simulink model "Controllo_din_inversa_OPERATIVO"  (R2023b)
settings: Solver=VariableStepAuto  StartTime=0.0  StopTime=10.0  RelTol=1e-3
undefined symbols (not defined in the file): b11, b12, b22, b_1, b_2, d_1, d_2, delta_b11, delta_b12, F1, F2, g1_1, g1_2, g2, gr, h, I_1, I_2, Im_1, Im_2, KD, KP, kr_1, kr_2, kt_1, kt_2, kv_1, kv_2, L_1, L_2, m_1, m_2, mm_2, qc_dd, Ra_1, Ra_2, tc, th1_0, th1d_0, th2_0, th2d_0
settings Model: Creator=Tommaso Savino  LastModifiedBy=Francesco_Savino

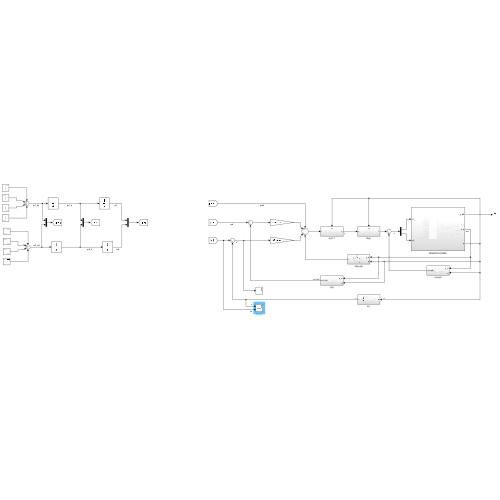
[thumbnail: Simulink's stored preview of the top-level diagram]
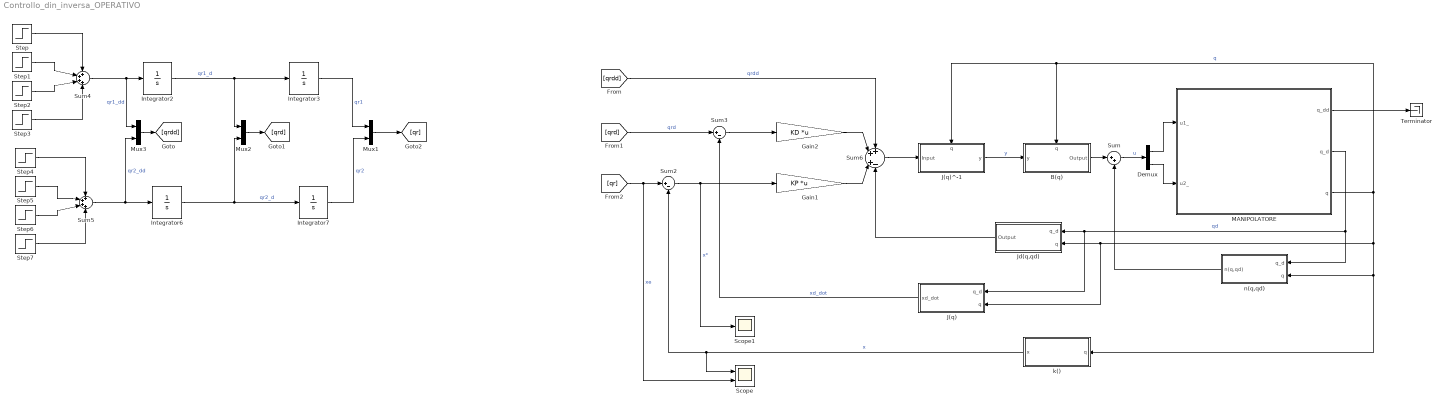
== system Controllo_din_inversa_OPERATIVO ==
  B(q) : Subsystem
      settings: PortSchema="{\"entries\":[{\"content\":{\"sides\":[{\"content\":{\"connectorIds\":[\"In1\"]},\"type\":\"ConnectorPlacement.EquallySpacedRectSide\",\"uuid\":\"bbc9a513-2d37-434b-b23e-4dc451bcd22f\"},{\"content\":{\"connectorIds\":[\"Out1\"],\"side\":\"RIGHT\"},\"type\":\"ConnectorPlacement.EquallySpacedRectSide\",\"uuid\":\"d2460926-2f38-42cc-bb12-745d42388ece\"},{\"content\":{\"connectorIds\":[\"In2\"],\"side\":\"TOP\"},\"type\":\"ConnectorPlacement.EquallySpacedRectSide\",\"uuid\":\"aeb2248f-89a4-438a-8c64-2b1b8cff1973\"}]},\"type\":\"ConnectorPlacement.EquallySpacedConnector\",\"uuid\":\"6c3609d5-174b-43d9-96a5-1a42f99e2581\"}],\"packageUris\":[\"http://schema.mathworks.com/mf0/Connector/R2020b\"],\"version\":\"1.0\"}"
  Demux : Demux  Outputs=2
  Gain1 : Gain  Gain=KP  Multiplication=Matrix(K*u) (u vector)
  Gain2 : Gain  Gain=KD  Multiplication=Matrix(K*u) (u vector)
  Integrator{2..3,6..7} (4 alike) : Integrator
  J(q) : Subsystem
  J(q)^-1 : Subsystem
      settings: PortSchema="{\"entries\":[{\"content\":{\"sides\":[{\"content\":{\"connectorIds\":[\"In1\"]},\"type\":\"ConnectorPlacement.EquallySpacedRectSide\",\"uuid\":\"515bc5bd-4876-4961-a034-aea24abec9fd\"},{\"content\":{\"connectorIds\":[\"Out1\"],\"side\":\"RIGHT\"},\"type\":\"ConnectorPlacement.EquallySpacedRectSide\",\"uuid\":\"1d0a2c9d-18e4-4c5e-8091-1d13b4417a11\"},{\"content\":{\"connectorIds\":[\"In2\"],\"side\":\"TOP\"},\"type\":\"ConnectorPlacement.EquallySpacedRectSide\",\"uuid\":\"0118a193-b043-45d6-8e6e-329b2fdaf764\"}]},\"type\":\"ConnectorPlacement.EquallySpacedConnector\",\"uuid\":\"91b6c9cd-145b-46ff-a2ec-d4d3d0262bff\"}],\"packageUris\":[\"http://schema.mathworks.com/mf0/Connector/R2020b\"],\"version\":\"1.0\"}"
  Jd(q,qd) : Subsystem
  MANIPOLATORE : Subsystem
  Mux1 : Mux  Inputs=2
  Mux2 : Mux  Inputs=2
  Mux3 : Mux  Inputs=2
  Scope : Scope  NumInputPorts=2
  Scope1 : Scope
  Step : Step  Time=0  After=qc_dd  SampleTime=0
  Step1 : Step  Time=tc  After=-qc_dd  SampleTime=0
  Step2 : Step  Time=tf-tc  After=-qc_dd  SampleTime=0
  Step3 : Step  Time=tf  After=qc_dd  SampleTime=0
  Step4 : Step  Time=0  After=qc_dd  SampleTime=0
  Step5 : Step  Time=tc  After=-qc_dd  SampleTime=0
  Step6 : Step  Time=tf-tc  After=-qc_dd  SampleTime=0
  Step7 : Step  Time=tf  After=qc_dd  SampleTime=0
  Sum : Sum  Inputs=|++
  Sum2 : Sum  Inputs=|+-
  Sum3 : Sum  Inputs=|+-
  Sum4 : Sum  Inputs=4
  Sum5 : Sum  Inputs=4
  Sum6 : Sum  Inputs=++|+-
  Terminator : Terminator
  k() : Subsystem
  n(q,qd) : Subsystem
  wires:
  Sum2/1 -> Scope1/1, Gain1/1  "x*"
  n(q,qd)/1(n(q,qd)) -> Sum/2
  Sum/1 -> Demux/1  "u"
  Gain1/1 -> Sum6/3
  MANIPOLATORE/2(q_d) -> n(q,qd)/1(q_d), J(q)/1(q_d), Jd(q,qd)/1(q_d)  "qd"
  Demux/2 -> MANIPOLATORE/2(u2_)
  MANIPOLATORE/1(q_dd) -> Terminator/1
  Demux/1 -> MANIPOLATORE/1(u1_)
  MANIPOLATORE/3(q) -> J(q)^-1/2(q), B(q)/2(q), J(q)/2(q), Jd(q,qd)/2(q), k()/1(q), n(q,qd)/2(q)  "q"
  Gain2/1 -> Sum6/2
  [qrdd] -> Sum6/1  "qrdd"
  Sum3/1 -> Gain2/1
  Step1/1 -> Sum4/2
  Step3/1 -> Sum4/4
  Step/1 -> Sum4/1
  Sum4/1 -> Mux3/1, Integrator2/1  "qr1_dd"
  Integrator2/1 -> Mux2/1, Integrator3/1  "qr1_d"
  Step2/1 -> Sum4/3
  Integrator3/1 -> Mux1/1  "qr1"
  Step7/1 -> Sum5/4
  Step6/1 -> Sum5/3
  Integrator6/1 -> Mux2/2, Integrator7/1  "qr2_d"
  Step5/1 -> Sum5/2
  Step4/1 -> Sum5/1
  Integrator7/1 -> Mux1/2  "qr2"
  Sum5/1 -> Mux3/2, Integrator6/1  "qr2_dd"
  Mux3/1 -> [qrdd]
  Mux2/1 -> [qrd]
  Mux1/1 -> [qr]
  [qrd] -> Sum3/1  "qrd"
  Sum6/1 -> J(q)^-1/1(Input)
  B(q)/1(Output) -> Sum/1
  J(q)/1(xd_dot) -> Sum3/2  "xd_dot"
  J(q)^-1/1(y) -> B(q)/1(y)  "y"
  [qr] -> Scope/2, Sum2/1  "xe"
  k()/1(x) -> Scope/1, Sum2/2  "x"
  Jd(q,qd)/1(Output) -> Sum6/4

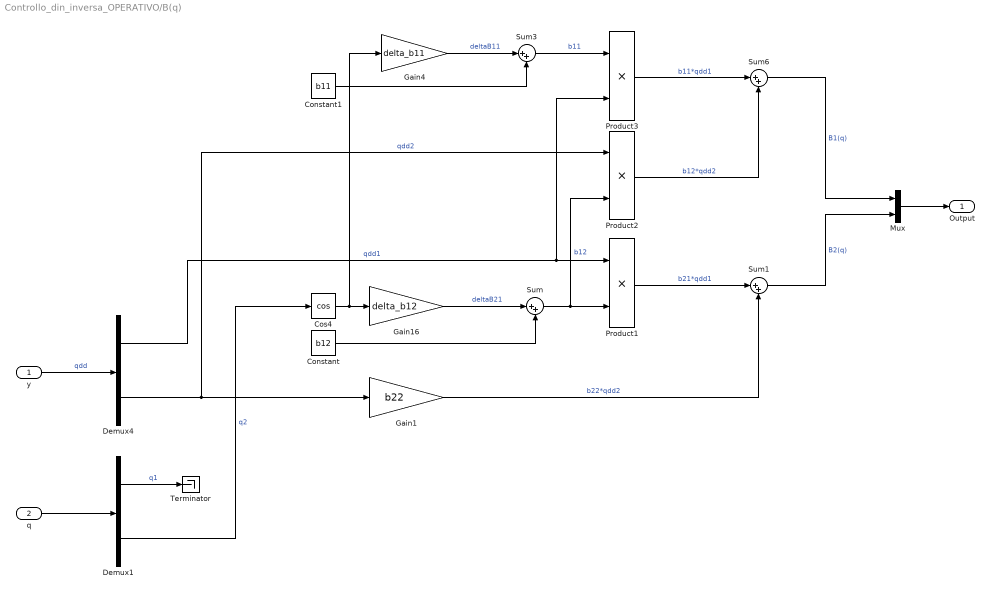
== system Controllo_din_inversa_OPERATIVO/B(q) ==
  y : Inport
  q : Inport  Port=2
  Constant : Constant  Value=b12
  Constant1 : Constant  Value=b11
  Cos4 : Trigonometry  Operator=cos
  Demux1 : Demux  Outputs=2
  Demux4 : Demux  Outputs=2
  Gain1 : Gain  Gain=b22
  Gain16 : Gain  Gain=delta_b12
  Gain4 : Gain  Gain=delta_b11
  Mux : Mux  Inputs=2
  Product1 : Product
  Product2 : Product
  Product3 : Product
  Sum{,1,3,6} (4 alike) : Sum  Inputs=|++
  Terminator : Terminator
  Output : Outport
  wires:
  Sum6/1 -> Mux/1  "B1(q)"
  Sum3/1 -> Product3/1  "b11"
  Constant1/1 -> Sum3/2
  Sum1/1 -> Mux/2  "B2(q)"
  Gain1/1 -> Sum1/2  "b22*qdd2"
  Product1/1 -> Sum1/1  "b21*qdd1"
  Sum/1 -> Product2/2, Product1/2  "b12"
  Constant/1 -> Sum/2
  Demux1/2 -> Cos4/1  "q2"
  Demux1/1 -> Terminator/1  "q1"
  Demux4/2 -> Product2/1, Gain1/1  "qdd2"
  Gain4/1 -> Sum3/1  "deltaB11"
  Demux4/1 -> Product1/1, Product3/2  "qdd1"
  Product3/1 -> Sum6/1  "b11*qdd1"
  Product2/1 -> Sum6/2  "b12*qdd2"
  Cos4/1 -> Gain4/1, Gain16/1
  Gain16/1 -> Sum/1  "deltaB21"
  y/1 -> Demux4/1  "qdd"
  q/1 -> Demux1/1
  Mux/1 -> Output/1

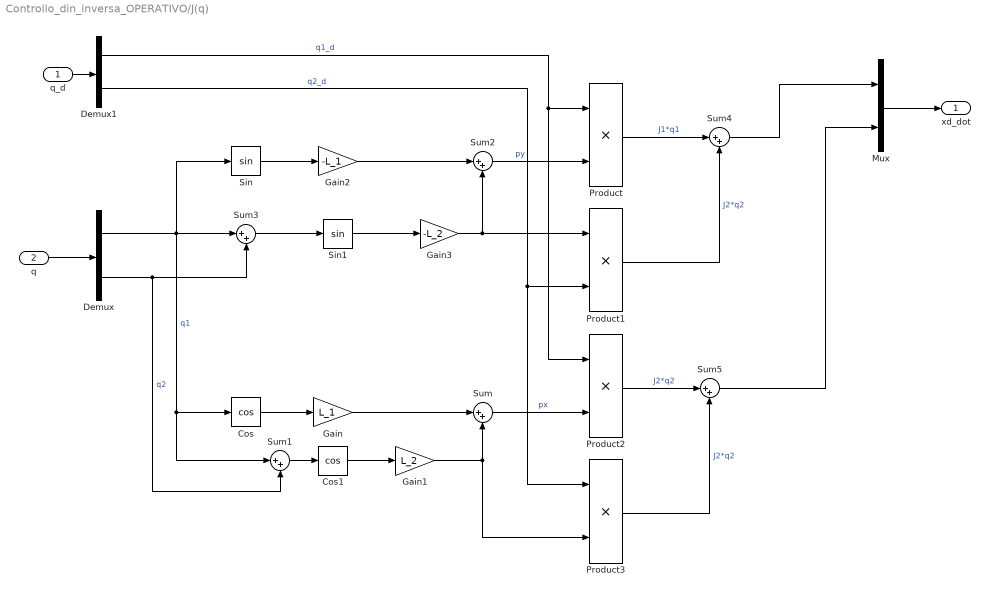
== system Controllo_din_inversa_OPERATIVO/J(q) ==
  q_d : Inport
  q : Inport  Port=2
  Cos : Trigonometry  Operator=cos
  Cos1 : Trigonometry  Operator=cos
  Demux : Demux  Outputs=2
  Demux1 : Demux  Outputs=2
  Gain : Gain  Gain=L_1
  Gain1 : Gain  Gain=L_2
  Gain2 : Gain  Gain=-L_1
  Gain3 : Gain  Gain=-L_2
  Mux : Mux  Inputs=2
  Product{,1..3} (4 alike) : Product
  Sin : Trigonometry
  Sin1 : Trigonometry
  Sum{,1..5} (6 alike) : Sum  Inputs=|++
  xd_dot : Outport
  wires:
  Sum3/1 -> Sin1/1
  Sin1/1 -> Gain3/1
  Sin/1 -> Gain2/1
  Sum2/1 -> Product/2  "py"
  Gain2/1 -> Sum2/1
  Gain3/1 -> Product1/1, Sum2/2
  q/1 -> Demux/1
  q_d/1 -> Demux1/1
  Demux1/1 -> Product2/1, Product/1  "q1_d"
  Product/1 -> Sum4/1  "J1*q1"
  Sum4/1 -> Mux/1
  Mux/1 -> xd_dot/1
  Demux1/2 -> Product3/1, Product1/2  "q2_d"
  Product1/1 -> Sum4/2  "J2*q2"
  Gain/1 -> Sum/1
  Cos1/1 -> Gain1/1
  Demux/1 -> Sum3/1, Cos/1, Sum1/1, Sin/1  "q1"
  Demux/2 -> Sum1/2, Sum3/2  "q2"
  Gain1/1 -> Product3/2, Sum/2
  Cos/1 -> Gain/1
  Sum1/1 -> Cos1/1
  Sum/1 -> Product2/2  "px"
  Product2/1 -> Sum5/1  "J2*q2"
  Product3/1 -> Sum5/2  "J2*q2"
  Sum5/1 -> Mux/2

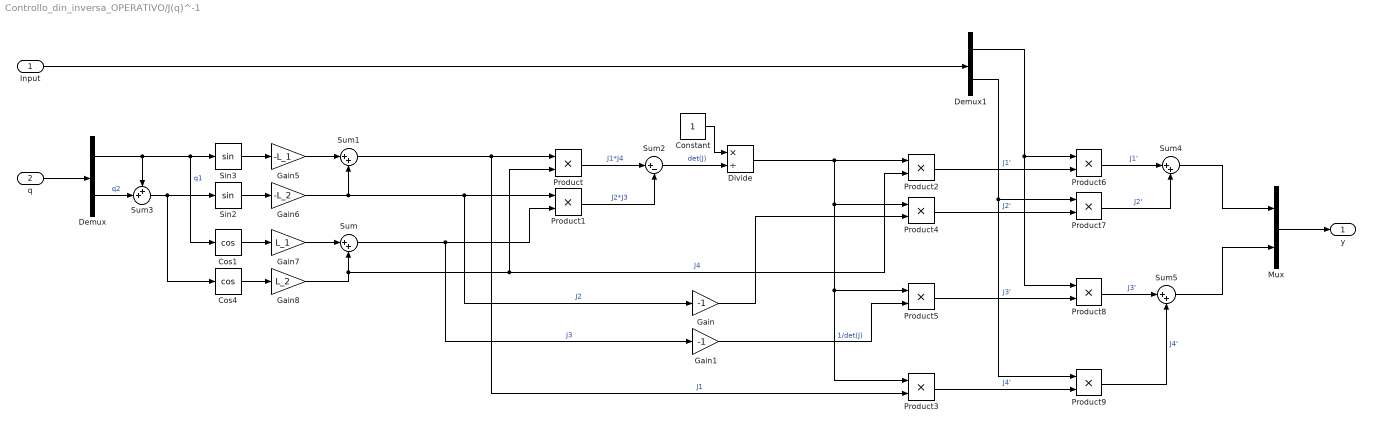
== system Controllo_din_inversa_OPERATIVO/J(q)^-1 ==
  Input : Inport
  q : Inport  Port=2
  Constant : Constant
  Cos1 : Trigonometry  Operator=cos
  Cos4 : Trigonometry  Operator=cos
  Demux : Demux  Outputs=2
  Demux1 : Demux  Outputs=2
  Divide : Product  Inputs=*/
  Gain : Gain  Gain=-1
  Gain1 : Gain  Gain=-1
  Gain5 : Gain  Gain=-L_1
  Gain6 : Gain  Gain=-L_2
  Gain7 : Gain  Gain=L_1
  Gain8 : Gain  Gain=L_2
  Mux : Mux  Inputs=2
  Product{,1..9} (10 alike) : Product
  Sin2 : Trigonometry
  Sin3 : Trigonometry
  Sum{,1,4..5} (4 alike) : Sum  Inputs=|++
  Sum2 : Sum  Inputs=|+-
  Sum3 : Sum  Inputs=++|
  y : Outport
  wires:
  Mux/1 -> y/1
  Input/1 -> Demux1/1
  Sin3/1 -> Gain5/1
  Demux/2 -> Sum3/2  "q2"
  Sum3/1 -> Sin2/1, Cos4/1
  Sin2/1 -> Gain6/1
  Gain7/1 -> Sum/1
  Gain5/1 -> Sum1/1
  Demux/1 -> Sin3/1, Cos1/1, Sum3/1  "q1"
  q/1 -> Demux/1
  Gain8/1 -> Product2/2, Product/2, Sum/2  "J4"
  Gain6/1 -> Gain/1, Product1/1, Sum1/2  "J2"
  Sum/1 -> Product1/2, Gain1/1  "J3"
  Sum1/1 -> Product3/2, Product/1  "J1"
  Cos1/1 -> Gain7/1
  Cos4/1 -> Gain8/1
  Product/1 -> Sum2/1  "J1*J4"
  Product1/1 -> Sum2/2  "J2*J3"
  Sum2/1 -> Divide/2  "det(J)"
  Constant/1 -> Divide/1
  Divide/1 -> Product5/1, Product3/1, Product4/1, Product2/1  "1/det(J)"
  Product2/1 -> Product6/2  "J1'"
  Product3/1 -> Product9/2  "J4'"
  Gain/1 -> Product4/2
  Product4/1 -> Product7/2  "J2'"
  Gain1/1 -> Product5/2
  Product5/1 -> Product8/2  "J3'"
  Product8/1 -> Sum5/1  "J3'"
  Product9/1 -> Sum5/2  "J4'"
  Product6/1 -> Sum4/1  "J1'"
  Product7/1 -> Sum4/2  "J2'"
  Sum4/1 -> Mux/1
  Sum5/1 -> Mux/2
  Demux1/1 -> Product8/1, Product6/1
  Demux1/2 -> Product9/1, Product7/1

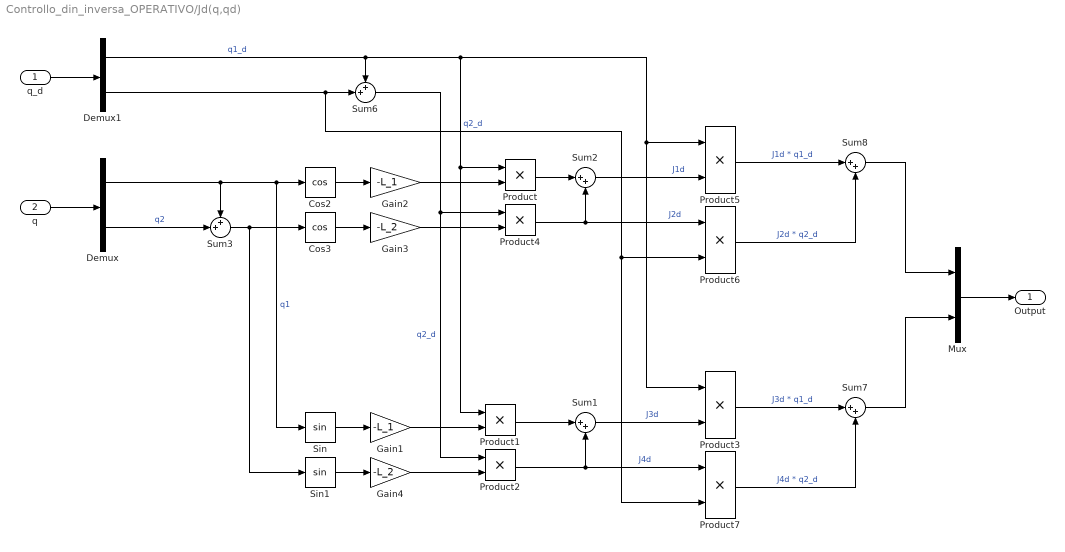
== system Controllo_din_inversa_OPERATIVO/Jd(q,qd) ==
  q_d : Inport
  q : Inport  Port=2
  Cos2 : Trigonometry  Operator=cos
  Cos3 : Trigonometry  Operator=cos
  Demux : Demux  Outputs=2
  Demux1 : Demux  Outputs=2
  Gain1 : Gain  Gain=-L_1
  Gain2 : Gain  Gain=-L_1
  Gain3 : Gain  Gain=-L_2
  Gain4 : Gain  Gain=-L_2
  Mux : Mux  Inputs=2
  Product{,1..7} (8 alike) : Product
  Sin : Trigonometry
  Sin1 : Trigonometry
  Sum{1..2,7..8} (4 alike) : Sum  Inputs=|++
  Sum3 : Sum  Inputs=++|
  Sum6 : Sum  Inputs=++|
  Output : Outport
  wires:
  Mux/1 -> Output/1
  q_d/1 -> Demux1/1
  q/1 -> Demux/1
  Gain3/1 -> Product4/2
  Gain2/1 -> Product/2
  Cos2/1 -> Gain2/1
  Cos3/1 -> Gain3/1
  Product/1 -> Sum2/1
  Sum3/1 -> Sin1/1, Cos3/1
  Product4/1 -> Product6/1, Sum2/2  "J2d"
  Sum6/1 -> Product2/1, Product4/1  "q2_d"
  Sum2/1 -> Product5/2  "J1d"
  Product5/1 -> Sum8/1  "J1d * q1_d"
  Product1/1 -> Sum1/1
  Demux1/2 -> Product7/2, Product6/2, Sum6/2  "q2_d"
  Sin/1 -> Gain1/1
  Demux/2 -> Sum3/2  "q2"
  Demux/1 -> Sin/1, Cos2/1, Sum3/1  "q1"
  Demux1/1 -> Product3/1, Product5/1, Product1/1, Product/1, Sum6/1  "q1_d"
  Sum1/1 -> Product3/2  "J3d"
  Gain4/1 -> Product2/2
  Product3/1 -> Sum7/1  "J3d * q1_d"
  Sin1/1 -> Gain4/1
  Gain1/1 -> Product1/2
  Product2/1 -> Product7/1, Sum1/2  "J4d"
  Product6/1 -> Sum8/2  "J2d * q2_d"
  Sum8/1 -> Mux/1
  Product7/1 -> Sum7/2  "J4d * q2_d"
  Sum7/1 -> Mux/2

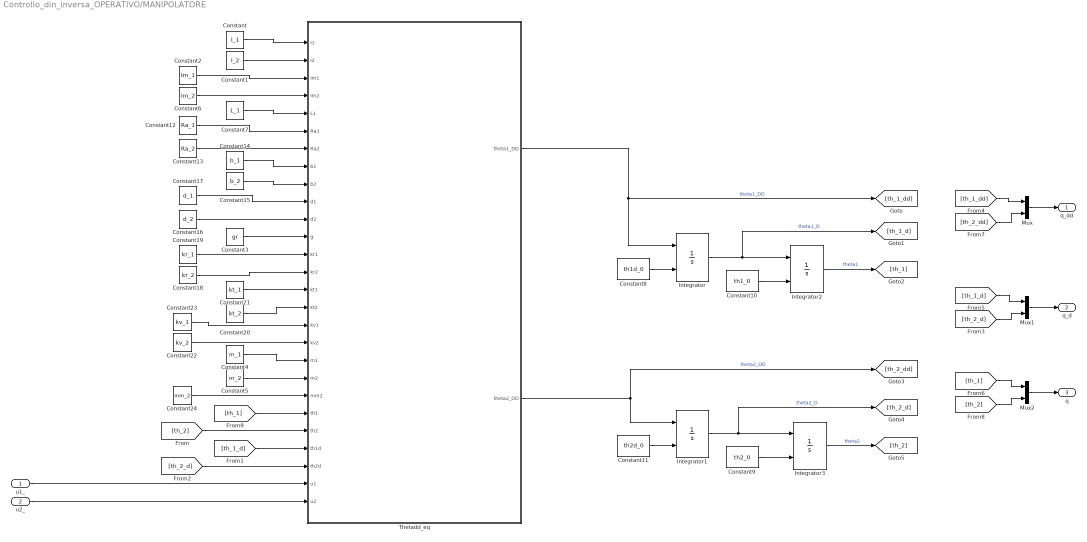
== system Controllo_din_inversa_OPERATIVO/MANIPOLATORE ==
  u1_ : Inport
  u2_ : Inport  Port=2
  Constant : Constant  Value=I_1
  Constant1 : Constant  Value=I_2
  Constant10 : Constant  Value=th1_0
  Constant11 : Constant  Value=th2d_0
  Constant12 : Constant  Value=Ra_1
  Constant13 : Constant  Value=Ra_2
  Constant14 : Constant  Value=b_1
  Constant15 : Constant  Value=b_2
  Constant16 : Constant  Value=d_2
  Constant17 : Constant  Value=d_1
  Constant18 : Constant  Value=kr_2
  Constant19 : Constant  Value=kr_1
  Constant2 : Constant  Value=Im_1
  Constant20 : Constant  Value=kt_2
  Constant21 : Constant  Value=kt_1
  Constant22 : Constant  Value=kv_2
  Constant23 : Constant  Value=kv_1
  Constant24 : Constant  Value=mm_2
  Constant3 : Constant  Value=gr
  Constant4 : Constant  Value=m_1
  Constant5 : Constant  Value=m_2
  Constant6 : Constant  Value=Im_2
  Constant7 : Constant  Value=L_1
  Constant8 : Constant  Value=th1d_0
  Constant9 : Constant  Value=th2_0
  Integrator{,1..3} (4 alike) : Integrator  InitialConditionSource=external
  Mux : Mux  Inputs=2
  Mux1 : Mux  Inputs=2
  Mux2 : Mux  Inputs=2
  Thetadd_eq : MATLAB Function  TreatAsAtomicUnit=on
  q_dd : Outport
  q_d : Outport  Port=2
  q : Outport  Port=3
  wires:
  Constant9/1 -> Integrator3/2
  Constant1/1 -> Thetadd_eq/2(I2)
  [th_2] -> Thetadd_eq/23(th2)
  Thetadd_eq/2(theta2_DD) -> Integrator1/1, [th_2_dd]  "theta2_DD"
  Constant5/1 -> Thetadd_eq/20(m2)
  Constant7/1 -> Thetadd_eq/5(L1)
  Constant3/1 -> Thetadd_eq/12(g)
  Thetadd_eq/1(theta1_DD) -> Integrator/1, [th_1_dd]  "theta1_DD"
  [th_1_d] -> Thetadd_eq/24(th1d)
  Integrator3/1 -> [th_2]  "theta2"
  Constant/1 -> Thetadd_eq/1(I1)
  Integrator2/1 -> [th_1]  "theta1"
  Constant2/1 -> Thetadd_eq/3(Im1)
  Integrator/1 -> [th_1_d], Integrator2/1  "theta1_D"
  Constant10/1 -> Integrator2/2
  Constant11/1 -> Integrator1/2
  Integrator1/1 -> [th_2_d], Integrator3/1  "theta2_D"
  Constant4/1 -> Thetadd_eq/19(m1)
  Constant8/1 -> Integrator/2
  [th_2_d] -> Thetadd_eq/25(th2d)
  Constant6/1 -> Thetadd_eq/4(Im2)
  u1_/1 -> Thetadd_eq/26(u1)
  u2_/1 -> Thetadd_eq/27(u2)
  [th_1_dd] -> Mux/1
  [th_2_dd] -> Mux/2
  Mux/1 -> q_dd/1
  [th_1_d] -> Mux1/1
  [th_2_d] -> Mux1/2
  Mux1/1 -> q_d/1
  [th_1] -> Mux2/1
  [th_2] -> Mux2/2
  Mux2/1 -> q/1
  Constant12/1 -> Thetadd_eq/6(Ra1)
  Constant13/1 -> Thetadd_eq/7(Ra2)
  Constant14/1 -> Thetadd_eq/8(b1)
  Constant15/1 -> Thetadd_eq/9(b2)
  Constant16/1 -> Thetadd_eq/11(d2)
  Constant17/1 -> Thetadd_eq/10(d1)
  Constant19/1 -> Thetadd_eq/13(kr1)
  Constant18/1 -> Thetadd_eq/14(kr2)
  Constant21/1 -> Thetadd_eq/15(kt1)
  Constant20/1 -> Thetadd_eq/16(kt2)
  Constant23/1 -> Thetadd_eq/17(kv1)
  Constant22/1 -> Thetadd_eq/18(kv2)
  Constant24/1 -> Thetadd_eq/21(mm2)
  [th_1] -> Thetadd_eq/22(th1)

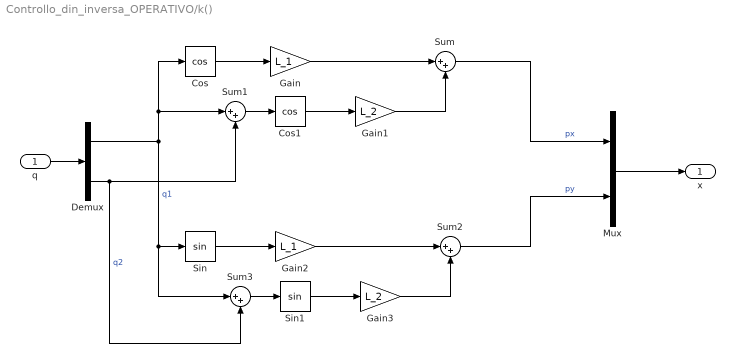
== system Controllo_din_inversa_OPERATIVO/k() ==
  q : Inport
  Cos : Trigonometry  Operator=cos
  Cos1 : Trigonometry  Operator=cos
  Demux : Demux  Outputs=2
  Gain : Gain  Gain=L_1
  Gain1 : Gain  Gain=L_2
  Gain2 : Gain  Gain=L_1
  Gain3 : Gain  Gain=L_2
  Mux : Mux  Inputs=2
  Sin : Trigonometry
  Sin1 : Trigonometry
  Sum{,1..3} (4 alike) : Sum  Inputs=|++
  x : Outport
  wires:
  q/1 -> Demux/1
  Demux/1 -> Sum3/1, Sin/1, Sum1/1, Cos/1  "q1"
  Demux/2 -> Sum1/2, Sum3/2  "q2"
  Cos/1 -> Gain/1
  Gain/1 -> Sum/1
  Sum1/1 -> Cos1/1
  Cos1/1 -> Gain1/1
  Gain1/1 -> Sum/2
  Sum3/1 -> Sin1/1
  Gain3/1 -> Sum2/2
  Sin/1 -> Gain2/1
  Sin1/1 -> Gain3/1
  Gain2/1 -> Sum2/1
  Sum2/1 -> Mux/2  "py"
  Sum/1 -> Mux/1  "px"
  Mux/1 -> x/1

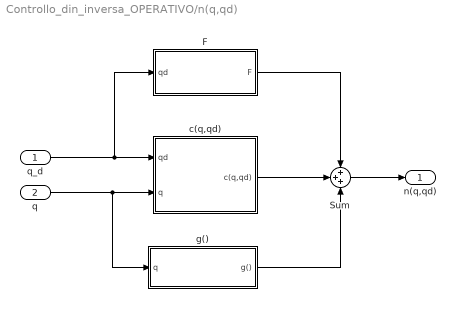
== system Controllo_din_inversa_OPERATIVO/n(q,qd) ==
  q_d : Inport
  q : Inport  Port=2
  F : Subsystem
  Sum : Sum  Inputs=+++
  c(q,qd) : Subsystem
  g() : Subsystem
  n(q,qd) : Outport
  wires:
  F/1(F) -> Sum/1
  q_d/1 -> c(q,qd)/1(qd), F/1(qd)
  Sum/1 -> n(q,qd)/1
  g()/1(g()) -> Sum/3
  c(q,qd)/1(c(q,qd)) -> Sum/2
  q/1 -> c(q,qd)/2(q), g()/1(q)

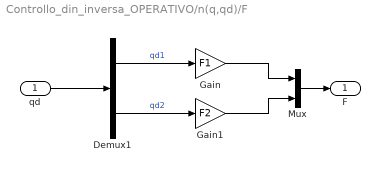
== system Controllo_din_inversa_OPERATIVO/n(q,qd)/F ==
  qd : Inport
  Demux1 : Demux  Outputs=2
  Gain : Gain  Gain=F1
  Gain1 : Gain  Gain=F2
  Mux : Mux  Inputs=2
  F : Outport
  wires:
  Demux1/2 -> Gain1/1  "qd2"
  Gain/1 -> Mux/1
  Mux/1 -> F/1
  Gain1/1 -> Mux/2
  qd/1 -> Demux1/1
  Demux1/1 -> Gain/1  "qd1"

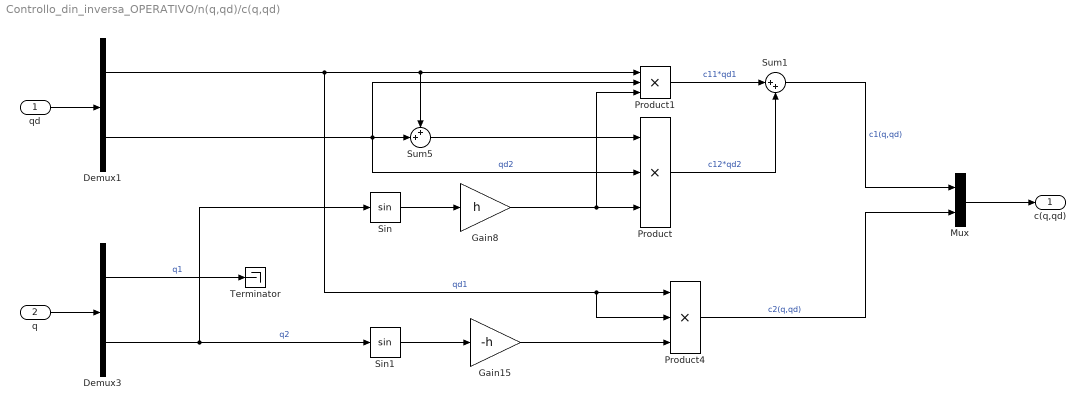
== system Controllo_din_inversa_OPERATIVO/n(q,qd)/c(q,qd) ==
  qd : Inport
  q : Inport  Port=2
  Demux1 : Demux  Outputs=2
  Demux3 : Demux  Outputs=2
  Gain15 : Gain  Gain=-h
  Gain8 : Gain  Gain=h
  Mux : Mux  Inputs=2
  Product : Product  Inputs=3
  Product1 : Product  Inputs=3
  Product4 : Product  Inputs=3
  Sin : Trigonometry
  Sin1 : Trigonometry
  Sum1 : Sum  Inputs=|++
  Sum5 : Sum  Inputs=++|
  Terminator : Terminator
  c(q,qd) : Outport
  wires:
  qd/1 -> Demux1/1
  q/1 -> Demux3/1
  Sin1/1 -> Gain15/1
  Gain15/1 -> Product4/3
  Sum1/1 -> Mux/1  "c1(q,qd)"
  Demux3/2 -> Sin/1, Sin1/1  "q2"
  Sum5/1 -> Product/1
  Product/1 -> Sum1/2  "c12*qd2"
  Demux1/2 -> Sum5/2, Product/2, Product1/2  "qd2"
  Sin/1 -> Gain8/1
  Demux1/1 -> Product4/1, Product4/2, Sum5/1, Product1/1  "qd1"
  Product1/1 -> Sum1/1  "c11*qd1"
  Product4/1 -> Mux/2  "c2(q,qd)"
  Demux3/1 -> Terminator/1  "q1"
  Gain8/1 -> Product/3, Product1/3
  Mux/1 -> c(q,qd)/1

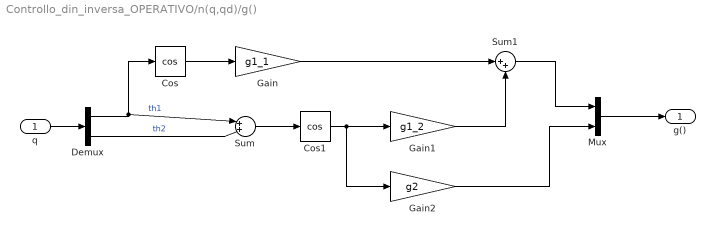
== system Controllo_din_inversa_OPERATIVO/n(q,qd)/g() ==
  q : Inport
  Cos : Trigonometry  Operator=cos
  Cos1 : Trigonometry  Operator=cos
  Demux : Demux  Outputs=2
  Gain : Gain  Gain=g1_1
  Gain1 : Gain  Gain=g1_2
  Gain2 : Gain  Gain=g2
  Mux : Mux  Inputs=2
  Sum : Sum  Inputs=|++|
  Sum1 : Sum  Inputs=|++
  g() : Outport
  wires:
  Gain2/1 -> Mux/2
  Mux/1 -> g()/1
  Sum1/1 -> Mux/1
  Gain1/1 -> Sum1/2
  Gain/1 -> Sum1/1
  Cos1/1 -> Gain1/1, Gain2/1
  Sum/1 -> Cos1/1
  Cos/1 -> Gain/1
  Demux/2 -> Sum/2  "th2"
  Demux/1 -> Sum/1, Cos/1  "th1"
  q/1 -> Demux/1

== matlab function Controllo_din_inversa_OPERATIVO/MANIPOLATORE/Thetadd_eq ==
  data: I1 input; theta1_DD output; I2 input; Im1 input; Im2 input; L1 input; Ra1 input; Ra2 input; b1 input; b2 input; d1 input; d2 input; g input; kr1 input; kr2 input; kt1 input; kt2 input; kv1 input; kv2 input; m1 input; m2 input; mm2 input; th1 input; th2 input; th1d input; th2d input; u1 input; u2 input; theta2_DD output
function [theta1_DD,theta2_DD] = Thetadd_eq(I1,I2,Im1,Im2,L1,Ra1,Ra2,b1,b2,d1,d2,g,kr1,kr2,kt1,kt2,kv1,kv2,m1,m2,mm2,th1,th2,th1d,th2d,u1,u2)
%#codegen

%    This function was generated by the Symbolic Math Toolbox version 23.2.
%    04-Mar-2024 11:53:02

% I1 = complex(I1);  % if required to enforce complex operations
% I2 = complex(I2);  % if required to enforce complex operations
% Im1 = complex(Im1);  % if required to enforce complex operations
% Im2 = complex(Im2);  % if required to enforce complex operations
% L1 = complex(L1);  % if required to enforce complex operations
% Ra1 = complex(Ra1);  % if required to enforce complex operations
% Ra2 = complex(Ra2);  % if required to enforce complex operations
% b1 = complex(b1);  % if required to enforce complex operations
% b2 = complex(b2);  % if required to enforce complex operations
% d1 = complex(d1);  % if required to enforce complex operations
% d2 = complex(d2);  % if required to enforce complex operations
% g = complex(g);  % if required to enforce complex operations
% kr1 = complex(kr1);  % if required to enforce complex operations
% kr2 = complex(kr2);  % if required to enforce complex operations
% kt1 = complex(kt1);  % if required to enforce complex operations
% kt2 = complex(kt2);  % if required to enforce complex operations
% kv1 = complex(kv1);  % if required to enforce complex operations
% kv2 = complex(kv2);  % if required to enforce complex operations
% m1 = complex(m1);  % if required to enforce complex operations
% m2 = complex(m2);  % if required to enforce complex operations
% mm2 = complex(mm2);  % if required to enforce complex operations
% th1 = complex(th1);  % if required to enforce complex operations
% th2 = complex(th2);  % if required to enforce complex operations
% th1d = complex(th1d);  % if required to enforce complex operations
% th2d = complex(th2d);  % if required to enforce complex operations
% u1 = complex(u1);  % if required to enforce complex operations
% u2 = complex(u2);  % if required to enforce complex operations
et1 = I2.*Ra1.*Ra2.*u1-I2.*Ra1.*Ra2.*u2-I2.*Ra1.*Ra2.*b1.*th1d+I2.*Ra1.*Ra2.*b2.*th2d-Im2.*Ra1.*Ra2.*kr2.*u2+Im2.*Ra1.*Ra2.*kr2.^2.*u1+Ra1.*Ra2.*d2.^2.*m2.*u1-Ra1.*Ra2.*d2.^2.*m2.*u2-Ra1.*Ra2.*b1.*d2.^2.*m2.*th1d+Ra1.*Ra2.*b2.*d2.^2.*m2.*th2d-I2.*Ra2.*kr1.^2.*kt1.*kv1.*th1d+I2.*Ra1.*kr2.^2.*kt2.*kv2.*th2d+Im2.*Ra1.*kr2.^3.*kt2.*kv2.*th2d+Im2.*Ra1.*Ra2.*b2.*kr2.*th2d-Im2.*Ra1.*Ra2.*b1.*kr2.^2.*th1d-L1.*Ra1.*Ra2.*d2.^2.*g.*m2.^2.*cos(th1)-I2.*L1.*Ra1.*Ra2.*g.*m2.*cos(th1)-I2.*L1.*Ra1.*Ra2.*g.*mm2.*cos(th1)-I2.*Ra1.*Ra2.*d1.*g.*m1.*cos(th1)-L1.*Ra1.*Ra2.*d2.*m2.*u2.*cos(th2);
et2 = L1.*Ra1.*Ra2.*d2.^3.*m2.^2.*th1d.^2.*sin(th2)+L1.*Ra1.*Ra2.*d2.^3.*m2.^2.*th2d.^2.*sin(th2)-Im2.*Ra2.*kr1.^2.*kr2.^2.*kt1.*kv1.*th1d-Ra2.*d2.^2.*kr1.^2.*kt1.*kv1.*m2.*th1d+Ra1.*d2.^2.*kr2.^2.*kt2.*kv2.*m2.*th2d-Im2.*L1.*Ra1.*Ra2.*g.*kr2.^2.*m2.*cos(th1)-Im2.*L1.*Ra1.*Ra2.*g.*kr2.^2.*mm2.*cos(th1)+I2.*L1.*Ra1.*Ra2.*d2.*m2.*th1d.^2.*sin(th2)+I2.*L1.*Ra1.*Ra2.*d2.*m2.*th2d.^2.*sin(th2)-Im2.*Ra1.*Ra2.*d1.*g.*kr2.^2.*m1.*cos(th1)-L1.*Ra1.*Ra2.*d2.^2.*g.*m2.*mm2.*cos(th1)-Ra1.*Ra2.*d1.*d2.^2.*g.*m1.*m2.*cos(th1)+Im2.*Ra1.*Ra2.*d2.*g.*kr2.*m2.*cos(th1+th2)+L1.*Ra1.*Ra2.*d2.^3.*m2.^2.*th1d.*th2d.*sin(th2).*2.0;
et3 = L1.*Ra1.*Ra2.*d2.^2.*g.*m2.^2.*cos(th1+th2).*cos(th2)+L1.*Ra1.*Ra2.*b2.*d2.*m2.*th2d.*cos(th2)+L1.^2.*Ra1.*Ra2.*d2.^2.*m2.^2.*th1d.^2.*cos(th2).*sin(th2)-Im2.*Ra1.*Ra2.*d2.*g.*kr2.^2.*m2.*cos(th1+th2)+I2.*L1.*Ra1.*Ra2.*d2.*m2.*th1d.*th2d.*sin(th2).*2.0+Im2.*L1.*Ra1.*Ra2.*d2.*kr2.*m2.*th1d.^2.*sin(th2)+L1.*Ra1.*d2.*kr2.^2.*kt2.*kv2.*m2.*th2d.*cos(th2)+Im2.*L1.*Ra1.*Ra2.*d2.*kr2.^2.*m2.*th2d.^2.*sin(th2)+Im2.*L1.*Ra1.*Ra2.*d2.*kr2.^2.*m2.*th1d.*th2d.*sin(th2).*2.0;
et4 = 1.0./(Ra1.*Ra2.*(I1.*I2+I2.*Im2-I2.*Im2.*kr2.*2.0+L1.^2.*d2.^2.*m2.^2+I2.*Im1.*kr1.^2+I1.*Im2.*kr2.^2+I2.*Im2.*kr2.^2+I2.*L1.^2.*m2+I2.*L1.^2.*mm2+I2.*d1.^2.*m1+I1.*d2.^2.*m2+Im2.*d2.^2.*m2-Im2.*d2.^2.*kr2.*m2.*2.0+Im1.*Im2.*kr1.^2.*kr2.^2+Im2.*L1.^2.*kr2.^2.*m2+Im2.*L1.^2.*kr2.^2.*mm2+Im1.*d2.^2.*kr1.^2.*m2+Im2.*d1.^2.*kr2.^2.*m1+Im2.*d2.^2.*kr2.^2.*m2+L1.^2.*d2.^2.*m2.*mm2+d1.^2.*d2.^2.*m1.*m2-L1.^2.*d2.^2.*m2.^2.*cos(th2).^2-Im2.*L1.*d2.*kr2.*m2.*cos(th2).*2.0+Im2.*L1.*d2.*kr2.^2.*m2.*cos(th2).*2.0));
et5 = et1+et2+et3;
theta1_DD = et4.*et5;
if nargout > 1
    et6 = -I1.*Ra1.*Ra2.*u2+I2.*Ra1.*Ra2.*u1-I2.*Ra1.*Ra2.*u2-Im2.*Ra1.*Ra2.*u2-I2.*Ra1.*Ra2.*b1.*th1d+I1.*Ra1.*Ra2.*b2.*th2d+I2.*Ra1.*Ra2.*b2.*th2d+Im2.*Ra1.*Ra2.*b2.*th2d+Im2.*Ra1.*Ra2.*kr2.*u1-Im1.*Ra1.*Ra2.*kr1.^2.*u2-L1.^2.*Ra1.*Ra2.*m2.*u2-L1.^2.*Ra1.*Ra2.*mm2.*u2-Ra1.*Ra2.*d1.^2.*m1.*u2+Ra1.*Ra2.*d2.^2.*m2.*u1-Ra1.*Ra2.*d2.^2.*m2.*u2-Ra1.*Ra2.*b1.*d2.^2.*m2.*th1d+Ra1.*Ra2.*b2.*d1.^2.*m1.*th2d+Ra1.*Ra2.*b2.*d2.^2.*m2.*th2d-I2.*Ra2.*kr1.^2.*kt1.*kv1.*th1d+I1.*Ra1.*kr2.^2.*kt2.*kv2.*th2d+I2.*Ra1.*kr2.^2.*kt2.*kv2.*th2d+Im2.*Ra1.*kr2.^2.*kt2.*kv2.*th2d-Im2.*Ra1.*Ra2.*b1.*kr2.*th1d;
    et7 = Im1.*Ra1.*Ra2.*b2.*kr1.^2.*th2d+L1.^2.*Ra1.*Ra2.*b2.*m2.*th2d+L1.^2.*Ra1.*Ra2.*b2.*mm2.*th2d-L1.*Ra1.*Ra2.*d2.^2.*g.*m2.^2.*cos(th1)+I1.*Ra1.*Ra2.*d2.*g.*m2.*cos(th1+th2)+Im2.*Ra1.*Ra2.*d2.*g.*m2.*cos(th1+th2)-I2.*L1.*Ra1.*Ra2.*g.*m2.*cos(th1)-I2.*L1.*Ra1.*Ra2.*g.*mm2.*cos(th1)-I2.*Ra1.*Ra2.*d1.*g.*m1.*cos(th1)+L1.*Ra1.*Ra2.*d2.*m2.*u1.*cos(th2)-L1.*Ra1.*Ra2.*d2.*m2.*u2.*cos(th2).*2.0-Im2.*Ra2.*kr1.^2.*kr2.*kt1.*kv1.*th1d+L1.*Ra1.*Ra2.*d2.^3.*m2.^2.*th1d.^2.*sin(th2)+L1.^3.*Ra1.*Ra2.*d2.*m2.^2.*th1d.^2.*sin(th2)+L1.*Ra1.*Ra2.*d2.^3.*m2.^2.*th2d.^2.*sin(th2)+Im1.*Ra1.*kr1.^2.*kr2.^2.*kt2.*kv2.*th2d+L1.^2.*Ra1.*kr2.^2.*kt2.*kv2.*m2.*th2d;
    et8 = L1.^2.*Ra1.*kr2.^2.*kt2.*kv2.*mm2.*th2d+L1.^2.*Ra1.*Ra2.*d2.*g.*m2.^2.*cos(th1+th2)-Ra2.*d2.^2.*kr1.^2.*kt1.*kv1.*m2.*th1d+Ra1.*d1.^2.*kr2.^2.*kt2.*kv2.*m1.*th2d+Ra1.*d2.^2.*kr2.^2.*kt2.*kv2.*m2.*th2d+L1.^2.*Ra1.*Ra2.*d2.*g.*m2.*mm2.*cos(th1+th2)+Ra1.*Ra2.*d1.^2.*d2.*g.*m1.*m2.*cos(th1+th2)+I1.*L1.*Ra1.*Ra2.*d2.*m2.*th1d.^2.*sin(th2)+I2.*L1.*Ra1.*Ra2.*d2.*m2.*th1d.^2.*sin(th2)+I2.*L1.*Ra1.*Ra2.*d2.*m2.*th2d.^2.*sin(th2)+Im2.*L1.*Ra1.*Ra2.*d2.*m2.*th1d.^2.*sin(th2)-L1.*Ra1.*Ra2.*d2.^2.*g.*m2.*mm2.*cos(th1)-Ra1.*Ra2.*d1.*d2.^2.*g.*m1.*m2.*cos(th1)-Im2.*Ra1.*Ra2.*d2.*g.*kr2.*m2.*cos(th1+th2)+L1.^3.*Ra1.*Ra2.*d2.*m2.*mm2.*th1d.^2.*sin(th2);
    et9 = L1.*Ra1.*Ra2.*d2.^3.*m2.^2.*th1d.*th2d.*sin(th2).*2.0-Im2.*L1.*Ra1.*Ra2.*g.*kr2.*m2.*cos(th1)-Im2.*L1.*Ra1.*Ra2.*g.*kr2.*mm2.*cos(th1)-Im2.*Ra1.*Ra2.*d1.*g.*kr2.*m1.*cos(th1)+L1.*Ra1.*Ra2.*d2.^2.*g.*m2.^2.*cos(th1+th2).*cos(th2)-L1.*Ra1.*Ra2.*b1.*d2.*m2.*th1d.*cos(th2)+L1.*Ra1.*Ra2.*b2.*d2.*m2.*th2d.*cos(th2).*2.0+L1.^2.*Ra1.*Ra2.*d2.^2.*m2.^2.*th1d.^2.*cos(th2).*sin(th2).*2.0+L1.^2.*Ra1.*Ra2.*d2.^2.*m2.^2.*th2d.^2.*cos(th2).*sin(th2)-L1.^2.*Ra1.*Ra2.*d2.*g.*m2.^2.*cos(th1).*cos(th2)+Im1.*Ra1.*Ra2.*d2.*g.*kr1.^2.*m2.*cos(th1+th2)-L1.^2.*Ra1.*Ra2.*d2.*g.*m2.*mm2.*cos(th1).*cos(th2)+L1.*Ra1.*Ra2.*d1.^2.*d2.*m1.*m2.*th1d.^2.*sin(th2);
    et10 = I2.*L1.*Ra1.*Ra2.*d2.*m2.*th1d.*th2d.*sin(th2).*2.0+Im2.*L1.*Ra1.*Ra2.*d2.*kr2.*m2.*th2d.^2.*sin(th2)-L1.*Ra2.*d2.*kr1.^2.*kt1.*kv1.*m2.*th1d.*cos(th2)+L1.*Ra1.*d2.*kr2.^2.*kt2.*kv2.*m2.*th2d.*cos(th2).*2.0+L1.^2.*Ra1.*Ra2.*d2.^2.*m2.^2.*th1d.*th2d.*cos(th2).*sin(th2).*2.0+Im1.*L1.*Ra1.*Ra2.*d2.*kr1.^2.*m2.*th1d.^2.*sin(th2)-L1.*Ra1.*Ra2.*d1.*d2.*g.*m1.*m2.*cos(th1).*cos(th2)+Im2.*L1.*Ra1.*Ra2.*d2.*kr2.*m2.*th1d.*th2d.*sin(th2).*2.0;
    et11 = 1.0./(Ra1.*Ra2.*(I1.*I2+I2.*Im2-I2.*Im2.*kr2.*2.0+L1.^2.*d2.^2.*m2.^2+I2.*Im1.*kr1.^2+I1.*Im2.*kr2.^2+I2.*Im2.*kr2.^2+I2.*L1.^2.*m2+I2.*L1.^2.*mm2+I2.*d1.^2.*m1+I1.*d2.^2.*m2+Im2.*d2.^2.*m2-Im2.*d2.^2.*kr2.*m2.*2.0+Im1.*Im2.*kr1.^2.*kr2.^2+Im2.*L1.^2.*kr2.^2.*m2+Im2.*L1.^2.*kr2.^2.*mm2+Im1.*d2.^2.*kr1.^2.*m2+Im2.*d1.^2.*kr2.^2.*m1+Im2.*d2.^2.*kr2.^2.*m2+L1.^2.*d2.^2.*m2.*mm2+d1.^2.*d2.^2.*m1.*m2-L1.^2.*d2.^2.*m2.^2.*cos(th2).^2-Im2.*L1.*d2.*kr2.*m2.*cos(th2).*2.0+Im2.*L1.*d2.*kr2.^2.*m2.*cos(th2).*2.0));
    et12 = -(et6+et7+et8+et9+et10);
    theta2_DD = et11.*et12;
end
end
